simulink model "Citation_2015a"  (R2015a)
settings: Solver=ode5  StartTime=0.0  StopTime=inf  FixedStep=0.01  RelTol=1e-3
InitFcn:
  | initcit
values from neighbouring files (symbols this model uses):
  aeroinit = [dp_ini;inicoef('CX0');inicoef('CXa');inicoef('CXa2');inicoef('CXq')     ;inicoef('CXde');inicoef('CY0');inicoef('CYB');inicoef('CYp');inicoef('CYr')     ;inicoef('CYda');inicoef('CYdr');inicoef('CZ0');inicoef('CZa');inicoef('CZq')     ;inicoef('CZde');inicoef('Cl0');inicoef('ClB');inicoef('Clp');inicoef('Clr')     ;inicoef('Clda');inicoef('Cldr');inicoef('Cm0');inicoef('Cma');inicoef('Cmq')     ; ...(+113 chars)    [initcit.m]
  Clda_thresh = 3.410e-2/2    (= 0.01705)    [initcit.m]
  h_l_old = zeros(6,sample_size)    [initcit.m]
  h_m_old = zeros(4,sample_size)    [initcit.m]
  h_n_old = zeros(6,sample_size)    [initcit.m]
  h_X_old = zeros(5,sample_size)    [initcit.m]
  h_Y_old = zeros(6,sample_size)    [initcit.m]
  h_Z_old = zeros(4,sample_size)    [initcit.m]
  I = [massinit(5),0, -massinit(8);0, massinit(6),0;-massinit(8),0, massinit(7)]    [initcit.m]
  p_l = [inicoef('Cl0');inicoef('ClB');inicoef('Clp');inicoef('Clr')     ;inicoef('Clda');inicoef('Cldr')].*ones(6,sample_size)    [initcit.m]
  p_m = [inicoef('Cm0');inicoef('Cma');inicoef('Cmq')     ;inicoef('Cmde')].*ones(4,sample_size)    [initcit.m]
  p_n = [inicoef('Cn0');inicoef('CnB');inicoef('Cnp');inicoef('Cnr')     ;inicoef('Cnda');inicoef('Cndr')].*ones(6,sample_size)    [initcit.m]
  p_X = [inicoef('CX0');inicoef('CXa');inicoef('CXa2');inicoef('CXq')     ;inicoef('CXde')].*ones(5,sample_size)    [initcit.m]
  p_Y = [inicoef('CY0');inicoef('CYB');inicoef('CYp');inicoef('CYr')     ;inicoef('CYda');inicoef('CYdr')].*ones(6,sample_size)    [initcit.m]
  p_Z = [inicoef('CZ0');inicoef('CZa');inicoef('CZq')     ;inicoef('CZde')].*ones(4,sample_size)    [initcit.m]
  Pcov_l = 10000*eye(6)    [initcit.m]
  Pcov_m = 10000*eye(4)    [initcit.m]
  Pcov_n = 10000*eye(6)    [initcit.m]
  Pcov_X = 10000*eye(5)    [initcit.m]
  Pcov_Y = 10000*eye(6)    [initcit.m]
  Pcov_Z = 10000*eye(4)    [initcit.m]
  replay = 0    [initcit.m]
  T0 = 288.15    [rho_test.m]
  timeend = inputsim.data{1}.Values.Time(end)    [initcit.m]
  Vw915 = 0    [initcit.m]
  winddir = 45*(pi/180)    (= 0.785398163397)    [initcit.m]
  x0 = []    [cessnac550_3d_sfnc.m]    (also in sfunxyauto.m)
  y_l = zeros(1,sample_size)    [initcit.m]
  y_l_est_old = zeros(size(y_l))    [initcit.m]
  y_m = zeros(1,sample_size)    [initcit.m]
  y_m_est_old = zeros(size(y_m))    [initcit.m]
  y_n = zeros(1,sample_size)    [initcit.m]
  y_n_est_old = zeros(size(y_n))    [initcit.m]
  y_X = zeros(1,sample_size)    [initcit.m]
  y_X_est_old = zeros(size(y_X))    [initcit.m]
  y_Y = zeros(1,sample_size)    [initcit.m]
  y_Y_est_old = zeros(size(y_Y))    [initcit.m]
  y_Z = zeros(1,sample_size)    [initcit.m]
  y_Z_est_old = zeros(size(y_Z))    [initcit.m]
undefined symbols (not defined in the file or in its folder): chord, cv1, cv2, cv3, cv4, deltagmax1, deltagmax2, deltagmax3, deltagmax4, Deng, ealphag, ealphas, g0, hDME, hGS, kt1, kt2, kt3, lh, massinit, matbuaf, matdaf, matdam, matdbbf, matdeaf, matdgaf, matdqaf, matduaf, matdwaw, matedhr, mateif, matelhr, matemhr, matemv1, matemv2, matemve, matetam, mateuaf, matfaaf, matfaxl, matff, matibaf, matibmh, matipaf, matipmh, matiraf, matiuaf, matiwaf, matlaf, matlam, matleaf, matleam, matlgaf, matlqaf, matluaf, matmaaf, matmaam, matmaf, matmam, matmbbf ... (+74)
undefined symbols (not defined in the file): matibb
libraries: simulink x13, templibrary x6, vrlib x1
(part 1 of 7)
settings Model: ExtModeTrigMode=oneshot  ExtModeArmWhenConnect=off  Creator=laurensvaneykeren  LastModifiedBy=Jelle
settings DataIOCC: LimitDataPoints=off  SignalLoggingName=sigsOut
settings OptimizationCC: BooleanDataType=off  ExpressionDepthLimit=2147483647
settings DebuggingCC: SaveWithParameterizedLinksMsg=none  UnderspecifiedInitializationDetection=Classic  MergeDetectMultiDrivingBlocksExec=none  SignalResolutionControl=TryResolveAllWithWarning  MultiTaskDSMMsg=warning  MultiTaskCondExecSysMsg=none  FcnCallInpInsideContextMsg=EnableAllAsWarning  StateNameClashWarn=warning
settings HardwareCC: TargetUnknown=on
settings RTWCC: SystemTargetFile=grt_malloc.tlc  GenCodeOnly=on  TemplateMakefile=grt_malloc_default_tmf
settings GRTTargetCC: GeneratePreprocessorConditionals=Use local settings  CombineOutputUpdateFcns=off  GRTInterface=on  UseMalloc=on

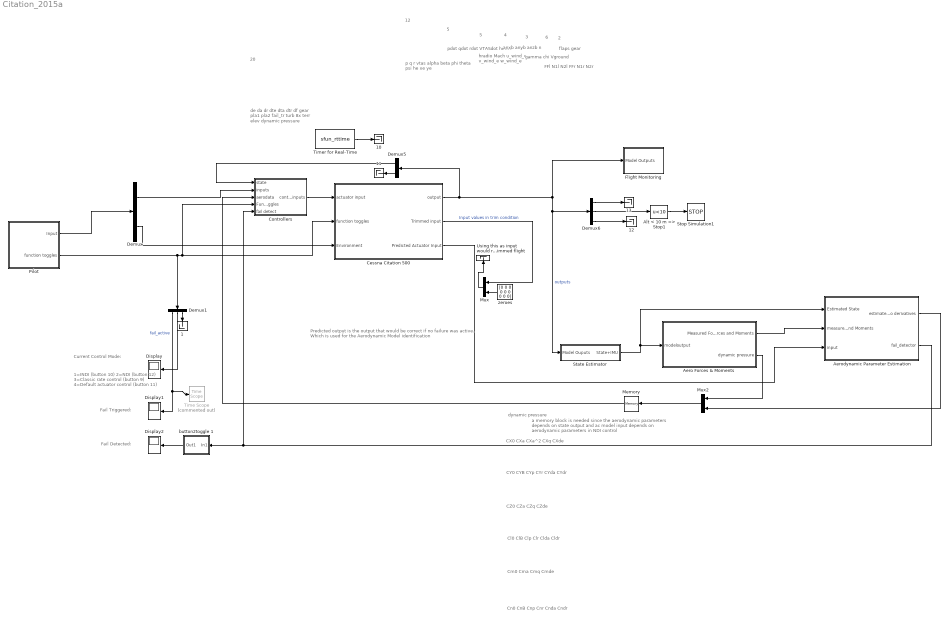
== system Citation_2015a ==
  note: a memory block is needed since the aerodynamic parameters depends on state output and ac model input depends on aerodynamic parameters in NDI control
  note: Predicted output is the output that would be correct if no failure was active.
      | Which is used for the Aerodynamic Model identification
  note: de
      | da
      | dr
      | dte
      | dta
      | dtr
      | df
      | gear
      | pla1
      | pla2
      | fail_tr
      | turb 8x
      | terr elev
      | dynamic pressure
  note: p
      | q
      | r
      | vtas
      | alpha
      | beta
      | phi
      | theta
      | psi
      | he
      | xe
      | ye
  note: pdot
      | qdot
      | rdot
      | VTASdot
      | hedot
  note: hradio
      | Mach
      | u_wind_e
      | v_wind_e
      | w_wind_e
  note: anxb
      | anyb
      | anzb
      | n
  note: gamma
      | chi
      | Vground
  note: flaps
      | gear
  note: FFl
      | N1l
      | N2l
      | FFr
      | N1r
      | N2r
  note: 12
  note: 5
  note: 5
  note: 4
  note: 3
  note: 6
  note: 2
  note: 20
  note: Cn0
      | CnB
      | Cnp
      | Cnr
      | Cnda
      | Cndr
  note: CZ0
      | CZa
      | CZq
      | CZde
  note: Cm0
      | Cma
      | Cmq
      | Cmde
  note: CY0
      | CYB
      | CYp
      | CYr
      | CYda
      | CYdr
  note: Cl0
      | ClB
      | Clp
      | Clr
      | Clda
      | Cldr
  note: CX0
      | CXa
      | CXa^2
      | CXq
      | CXde
  note: dynamic pressure
  note: Current Control Mode:
  note: 1=INDI (button 10)
      | 2=NDI (button 12)
      | 3=Classic rate control (button 9)
      | 4=Default actuator control (button 11)
  note: Fail Triggered:
  note: Fail Detected:
  {1,10..13} (5 alike) : Terminator
  "Aero Forces & Moments " : Subsystem
  Aerodynamic Parameter Estimation : Subsystem
  Alt < 10 m => Stop1 : Fcn  Expr=u<10
  Cessna Citation 500 : Subsystem  mask(Citation Aircraft Model){trimdatafile=example.tri}
      mask prompts: trimdatafile "Trim Condition"
      mask init:
      | initcit;
      mask Display:
      | image(imread('Citation.jpg'))
      | port_label('input', 1, 'Inputs')
      | port_label('input', 2, 'Function Toggles')
      | port_label('input', 3, 'Environment')
      | port_label('output', 1, 'Outputs')
      | port_label('output', 2, 'Trim inputs')
      | port_label('output', 3, 'Predicted control input')
  Controllers : Subsystem
  Demux : Demux  Outputs=[10 9]
  Demux1 : Demux  Outputs=[1 1 2]
  Demux5 : Demux  Outputs=[17 20]
  Demux6 : Demux  Outputs=[9 1 27]
  Display : Display
  Display1 : Display
  Display2 : Display
  Flight Monitoring : Subsystem
  Memory : Memory  X0=aeroinit
  Mux : Mux  Inputs=2
  Mux2 : Mux  Inputs=2
  Pilot : Subsystem
  "State Estimator " : Subsystem
  Stop Simulation1 : Stop
  Time Scope : TimeScope  Commented=on  DefaultConfigurationName=spbscopes.TimeScopeBlockCfg
  Timer for Real-Time : S-Function  FunctionName=sfun_rttime  Parameters=1  SFunctionDeploymentMode=off  EnableBusSupport=off
  Using this as input would result in trimmed flight : Terminator
  button2toggle 1 : Subsystem
  zeroes : Constant  Value=[0 0 0 0 0 0 0 0 0]
  wires:
  Demux/1 -> Controllers/2(inputs)
  Pilot/1(Input) -> Demux/1
  Cessna Citation 500/1(output) -> Demux6/1, "State Estimator "/1(Model Ouputs), Flight Monitoring/1(Model Outputs), Demux5/1  "outputs"
  Demux/2 -> Cessna Citation 500/3(Environment)
  Cessna Citation 500/2(Trimmed input) -> Mux/1  "Input values in trim condition"
  zeroes/1 -> Mux/2
  Mux/1 -> Using this as input would result in trimmed flight/1
  "State Estimator "/1(State+IMU) -> Aerodynamic Parameter Estimation/1("Estimated State "), "Aero Forces & Moments "/1(modeloutput)
  Cessna Citation 500/3(Predicted Actuator Input) -> Aerodynamic Parameter Estimation/3("input ")
  "Aero Forces & Moments "/1(Measured Forces and Moments) -> Aerodynamic Parameter Estimation/2("measured forces and Moments ")
  Aerodynamic Parameter Estimation/1(estimated aero derivatives) -> Mux2/2
  "Aero Forces & Moments "/2("dynamic pressure ") -> Mux2/1
  Mux2/1 -> Memory/1
  Memory/1 -> Controllers/3(aerodata)
  Timer for Real-Time/1 -> 10/1
  Aerodynamic Parameter Estimation/2(fail_detector) -> Controllers/5(fail detect), button2toggle 1/1(In1)
  Demux5/2 -> 11/1
  Demux5/1 -> Controllers/1(state)
  Controllers/1(control inputs) -> Cessna Citation 500/1(actuator input)
  Demux6/3 -> 12/1
  Demux6/1 -> 13/1
  Demux6/2 -> Alt < 10 m => Stop1/1
  Alt < 10 m => Stop1/1 -> Stop Simulation1/1
  Pilot/2(function toggles) -> Controllers/4("Function Toggles "), Cessna Citation 500/2("function toggles "), Demux1/1
  Demux1/1 -> Time Scope/1, Display1/1  "fail_active"
  Demux1/2 -> Display/1
  button2toggle 1/1(Out1) -> Display2/1
  Demux1/3 -> 1/1

== system Citation_2015a/Aero Forces & Moments  ==
  note: Kinematic Force Coeffient determination
  note: anxb
      | anyb
      | anzb
      | n
  note: hradio
      | Mach
      | u_wind_e
      | v_wind_e
      | w_wind_e
  note: p
      | q
      | r
      | vtas
      | alpha
      | beta
      | phi
      | theta
      | psi
      | he
      | xe
      | ye
  note: gamma
      | chi
      | Vground
  note: pdot
      | qdot
      | rdot
      | VTASdot
      | hedot
  note: FFl
      | N1l
      | N2l
      | FFr
      | N1r
      | N2r
  note: flaps
      | gear
  note: 6
  note: 5
  note: 12
  note: 3
  note: 5
  note: 4
  note: 2
  note: CX
      | CY
      | CZ
      | Cl
      | Cm
      | Cn
  modeloutput : Inport
  Aerodynamic Force Components : Subsystem
  Aerodynamic Moment Components : Subsystem
  Calculate Dynamic Pressure : Subsystem
  Mux : Mux  Inputs=2
  Measured Forces and Moments : Outport
  "dynamic pressure " : Outport  Port=2
  wires:
  Aerodynamic Force Components/1(Out1) -> Mux/1
  modeloutput/1 -> Calculate Dynamic Pressure/1(In1), Aerodynamic Moment Components/1("State "), Aerodynamic Force Components/1("model output ")
  Calculate Dynamic Pressure/1(Out1) -> "dynamic pressure "/1, Aerodynamic Moment Components/2("Dynamic Pressure "), Aerodynamic Force Components/2(dynamic pressure)
  Aerodynamic Moment Components/1(Out1) -> Mux/2
  Mux/1 -> Measured Forces and Moments/1

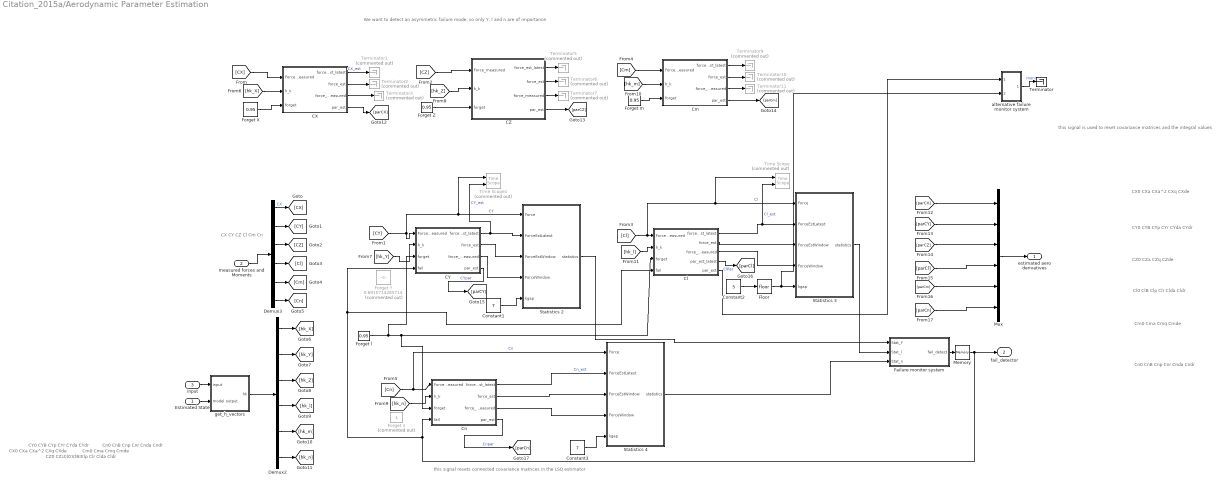
== system Citation_2015a/Aerodynamic Parameter Estimation ==
  note: this signal is used to reset covariance matrices and the integral values
  note: this signal resets connected covariance matrices in the LSQ estimator
  note: We want to detect an asymmetric failure mode, so only Y, l and n are of importance
  note: CX
      | CY
      | CZ
      | Cl
      | Cm
      | Cn
  note: Cm0
      | Cma
      | Cmq
      | Cmde
  note: Cn0
      | CnB
      | Cnp
      | Cnr
      | Cnda
      | Cndr
  note: CY0
      | CYB
      | CYp
      | CYr
      | CYda
      | CYdr
  note: CZ0
      | CZa
      | CZq
      | CZde
  note: CX0
      | CXa
      | CXa^2
      | CXq
      | CXde
  note: Cl0
      | ClB
      | Clp
      | Clr
      | Clda
      | Cldr
  note: Cl0
      | ClB
      | Clp
      | Clr
      | Clda
      | Cldr
  note: CY0
      | CYB
      | CYp
      | CYr
      | CYda
      | CYdr
  note: Cm0
      | Cma
      | Cmq
      | Cmde
  note: CX0
      | CXa
      | CXa^2
      | CXq
      | CXde
  note: CZ0
      | CZa
      | CZq
      | CZde
  note: Cn0
      | CnB
      | Cnp
      | Cnr
      | Cnda
      | Cndr
  "Estimated State " : Inport
  "measured forces and Moments " : Inport  Port=2
  "input " : Inport  Port=3
  CX : Subsystem
  CY : Subsystem
  CZ : Subsystem
  Cl : Subsystem
  Cm : Subsystem
  Cn : Subsystem
  Constant1 : Constant  Value=7
  Constant2 : Constant  Value=5
  Constant3 : Constant  Value=7
  Demux2 : Demux  Outputs=[5 6 4 6 4 6]
  Demux3 : Demux  Outputs=[1 1 1 1 1 1]
  "Failure monitor system " : Subsystem
  Floor : Rounding
  Forget X : Constant  Value=0.95
  Forget Y : Constant  Commented=on  Value=0.6910714285714
  Forget Z : Constant  Value=0.95
  Forget l : Constant  Value=0.95
  Forget m : Constant  Value=0.95
  Forget n : Constant  Commented=on
  Memory : Memory
  Mux : Mux  Inputs=6
  Statistics 2 : Subsystem
  Statistics 3 : Subsystem
  Statistics 4 : Subsystem
  Terminator : Terminator
  Terminator{1..3,5..7,9..11} (9 alike) : Terminator  Commented=on
  Time Scope : TimeScope  Commented=on  DefaultConfigurationName=spbscopes.TimeScopeBlockCfg  NumInputPorts=2
  Time Scope1 : TimeScope  Commented=on  DefaultConfigurationName=spbscopes.TimeScopeBlockCfg  NumInputPorts=2
  alternative failure monitor system : Subsystem
  get_h_vectors : Subsystem
  estimated aero derivatives : Outport
  fail_detector : Outport  Port=2
  wires:
  "input "/1 -> get_h_vectors/1(input)
  "Estimated State "/1 -> get_h_vectors/2(model output)
  get_h_vectors/1(hk) -> Demux2/1
  "measured forces and Moments "/1 -> Demux3/1
  Demux3/2 -> [CY]
  CX/4(par_est) -> [parCX]
  Forget X/1 -> CX/3(forget)
  Forget Z/1 -> CZ/3(forget)
  Forget l/1 -> CY/3(forget), Cn/3(forget), Cl/3(forget)
  Forget m/1 -> Cm/3(forget)
  CY/1(force_est_latest) -> Time Scope1/2, Statistics 2/2(ForceEstLatest)  "CY_est"
  CY/2(force_est) -> Statistics 2/3(ForceEstWindow)
  CY/3(force_measured) -> Statistics 2/4(ForceWindow)
  Constant1/1 -> Statistics 2/5("kgap ")
  Cl/1(force_est_latest) -> Time Scope/2, Statistics 3/2(ForceEstLatest)  "Cl_est"
  Cl/2(force_est) -> Statistics 3/3(ForceEstWindow)
  Cl/3(force_measured) -> Statistics 3/4(ForceWindow)
  Constant2/1 -> Floor/1
  Cn/1(force_est_latest) -> Statistics 4/2(ForceEstLatest)  "Cn_est"
  Cn/2(force_est) -> Statistics 4/3(ForceEstWindow)
  Constant3/1 -> Statistics 4/5("kgap ")
  Demux3/1 -> [CX]  "CX"
  [CX] -> CX/1(Force_measured)
  [CY] -> CY/1(Force_measured), Time Scope1/1, Statistics 2/1(Force)  "CY"
  Demux3/3 -> [CZ]
  [CZ] -> CZ/1(Force_measured)
  Demux3/4 -> [Cl]
  [Cl] -> Time Scope/1, Statistics 3/1(Force), Cl/1(Force_measured)  "Cl"
  Demux3/5 -> [Cm]
  [Cm] -> Cm/1(Force_measured)
  Demux3/6 -> [Cn]
  [Cn] -> Statistics 4/1(Force), Cn/1(Force_measured)  "Cn"
  Demux2/1 -> [hk_X]
  Demux2/2 -> [hk_Y]
  Demux2/3 -> [hk_Z]
  Demux2/4 -> [hk_l]
  Demux2/5 -> [hk_m]
  Demux2/6 -> [hk_n]
  [hk_X] -> CX/2(h_k)
  [hk_Y] -> CY/2(h_k)
  [hk_Z] -> CZ/2(h_k)
  [hk_l] -> Cl/2(h_k)
  [hk_m] -> Cm/2(h_k)
  [hk_n] -> Cn/2(h_k)
  Cn/3(force_measured) -> Statistics 4/4(ForceWindow)
  CX/1(force_est_latest) -> Terminator1/1  "CX_est"
  CX/2(force_est) -> Terminator2/1
  CX/3(force_measured) -> Terminator3/1
  CY/4(par_est) -> [parCY]  "CYpar"
  CZ/2(force_est) -> Terminator6/1
  CZ/3(force_measured) -> Terminator7/1
  CZ/1(force_est_latest) -> Terminator5/1
  Cm/1(force_est_latest) -> Terminator9/1
  Cm/2(force_est) -> Terminator10/1
  Cm/3(force_measured) -> Terminator11/1
  Cm/4(par_est) -> [parCm]
  Statistics 4/1(statistics) -> "Failure monitor system "/3(Stat_n)
  Statistics 3/1(statistics) -> "Failure monitor system "/2(Stat_l)
  Statistics 2/1(statistics) -> "Failure monitor system "/1(Stat_Y)
  CZ/4(par_est) -> [parCZ]
  Cl/4(par_est_latest) -> [parCl]  "ClPar"
  Cn/4(par_est) -> [parCn]  "Cnpar"
  [parCX] -> Mux/1
  [parCY] -> Mux/2
  [parCZ] -> Mux/3
  [parCl] -> Mux/4
  [parCm] -> Mux/5
  [parCn] -> Mux/6
  Mux/1 -> estimated aero derivatives/1
  Floor/1 -> alternative failure monitor system/2(In3), Statistics 3/5("kgap ")
  Cl/5(par_est) -> alternative failure monitor system/1(In2)
  "Failure monitor system "/1(fail_detect) -> Memory/1
  Memory/1 -> fail_detector/1, Cl/4("fail "), CY/4(fail), Cn/4("fail ")
  alternative failure monitor system/1(Out1) -> Terminator/1  "moni"

== system Citation_2015a/Cessna Citation 500 ==
  note: this is the actuator input that is always without failure
  note: p
      | q
      | r
      | vtas
      | alpha
      | beta
      | phi
      | theta
      | psi
      | he
      | xe
      | ye
  note: de
      | da
      | dr
      | dte
      | dta
      | dtr
      | df
      | gear
      | pla1
      | pla2
  note: pdot
      | qdot
      | rdot
      | VTASdot
      | hedot
  note: hradio
      | Mach
      | u_wind_e
      | v_wind_e
      | w_wind_e
  note: anxb
      | anyb
      | anzb
      | n
  note: gamma
      | chi
      | Vground
  note: turb 8x
      | terr_elev
  note: flaps
      | gear
  note: de
      | da
      | dr
      | dte
      | dta
      | dtr
      | df
      | gear
      | pla1
      | pla2
  note: FFl
      | N1l
      | N2l
      | FFr
      | N1r
      | N2r
  note: fail_aileron
  actuator input : Inport
  "function toggles " : Inport  Port=2
  Environment : Inport  Port=3
  Actuators : Subsystem
  Citation model DASMAT : Subsystem
  Control Inputs : TimeScope  Commented=on  DefaultConfigurationName=spbscopes.TimeScopeBlockCfg  NumInputPorts=3
  Demux : Demux  Outputs=[1 3]
  Demux1 : Demux  Outputs=[1 1 1 7]
  Demux4 : Demux  Outputs=[8 2]
  Gain : Gain  Commented=on  Gain=180/pi
  Gain1 : Gain  Commented=on  Gain=180/pi
  Gain2 : Gain  Commented=on  Gain=180/pi
  Mux1 : Mux  Inputs=7
  Mux2 : Mux  Inputs=2
  Terminator : Terminator
  Terminator1 : Terminator
  trim conditions : Subsystem
  ua sel : Selector  IndexOptions=Index vector (dialog)  Indices=[5 6]  OutputSizes=1
  xdot sel : Selector  IndexOptions=Index vector (dialog)  Indices=[1 2 3 4 10]  OutputSizes=1
  yacc sel : Selector  IndexOptions=Index vector (dialog)  Indices=[4 5 6 15]  OutputSizes=1
  yair sel : Selector  IndexOptions=Index vector (dialog)  Indices=[6 9 22 23 24]  OutputSizes=1
  yfp sel : Selector  IndexOptions=Index vector (dialog)  Indices=[1 2 15]  OutputSizes=1
  ypp sel : Selector  IndexOptions=Index vector (dialog)  Indices=[2 3 4 13 14 15]  OutputSizes=1
  output : Outport
  Trimmed input : Outport  Port=2
  Predicted Actuator Input : Outport  Port=3
  wires:
  Mux1/1 -> output/1
  Citation model DASMAT/1(x) -> Mux1/1
  Demux4/1 -> Citation model DASMAT/1(ua), ua sel/1
  Demux4/2 -> Citation model DASMAT/2(ut)
  Citation model DASMAT/3(yair) -> yair sel/1
  yair sel/1 -> Mux1/3
  Citation model DASMAT/2(xdot) -> xdot sel/1
  xdot sel/1 -> Mux1/2
  yacc sel/1 -> Mux1/4
  Citation model DASMAT/4(yacc) -> yacc sel/1
  yfp sel/1 -> Mux1/5
  Citation model DASMAT/5(yfp) -> yfp sel/1
  trim conditions/1(ua) -> Mux2/1
  trim conditions/2(ut) -> Mux2/2
  Mux2/1 -> Trimmed input/1
  ua sel/1 -> Mux1/7
  Citation model DASMAT/6(ypp) -> ypp sel/1
  ypp sel/1 -> Mux1/6
  Actuators/2(Actuator_pred) -> Predicted Actuator Input/1
  Environment/1 -> Citation model DASMAT/3(Environment)
  Demux1/1 -> Gain/1  "de true"
  Demux1/2 -> Gain1/1  "da true"
  Demux1/3 -> Gain2/1  "dr true"
  Demux1/4 -> Terminator/1
  actuator input/1 -> Actuators/1(In)  "actuator_input"
  Demux/1 -> Actuators/2("failure toggle ")
  "function toggles "/1 -> Demux/1
  Demux/2 -> Terminator1/1
  Actuators/1(Actuator_True) -> Demux1/1, Demux4/1
  Gain/1 -> Control Inputs/1
  Gain1/1 -> Control Inputs/2
  Gain2/1 -> Control Inputs/3

== system Citation_2015a/Controllers ==
  note: map joystick inputs to reference rotational rates
  note: This signal resets the integral values of all connected PIDs
      | Resets when manually changing the control mode and when failure state changes.
  note: 1=INDI (button 10)
      | 2=NDI (button 12)
      | 3=Classic rate control (button 9)
      | 4=Default actuator control (button 11)
  note: Aerodata Description
  note: [1]
  note: p
      | q
      | r
      | vtas
      | alpha
      | beta
      | phi
      | theta
      | psi
      | he
      | xe
      | ye
  note: de
      | da
      | dr
      | dte
      | dta
      | dtr
      | df
      | gear
      | pla1
      | pla2
  note: CX0
      | CXa
      | CXa^2
      | CXq
      | CXde
  note: Cm0
      | Cma
      | Cmq
      | Cmde
  note: CY0
      | CYB
      | CYp
      | CYr
      | CYda
      | CYdr
  note: CZ0
      | CZa
      | CZq
      | CZde
  note: Cn0
      | CnB
      | Cnp
      | Cnr
      | Cnda
      | Cndr
  note: dynamic pressure
  note: Cl0
      | ClB
      | Clp
      | Clr
      | Clda
      | Cldr
  note: [2:6]
  note: [7:12]
  note: [13:16]
  note: [17:22]
  note: [23:26]
  note: [27:32]
  state : Inport
  inputs : Inport  Port=2
  aerodata : Inport  Port=3
  "Function Toggles " : Inport  Port=4
  fail detect : Inport  Port=5
  "A/T " : Gain  Gain=[1 1 1 1 1 1 1 1 1 1]  SaturateOnIntegerOverflow=on  OutDataTypeStr=Inherit: Same as input  ParamDataTypeStr=Inherit: Same as input
  ANDI rotational rate controller : Subsystem
  Classical rotational rate control : Subsystem
  Constant : Constant
  Constant1 : Constant  Value=0
  Constant3 : Constant  Commented=on  Value=aeroinit
  Default Actuator Control : Subsystem
  Demux1 : Demux  Outputs=[12 5]
  Demux2 : Demux
  Display1 : Display
  Gain : Gain
  Generate Integral reset pulse : Subsystem
  INDI rotational rate controller : Subsystem
  Input to omega_ref (Beta feedback included) : Subsystem
  Memory : Memory  X0=zeros(5,1)
  Multiply : Product
  Multiport Switch : MultiPortSwitch  Inputs=4
  Switch : Switch  Criteria=u2 > Threshold
  Terminator1 : Terminator
  add controller outputs to pilot inputs : Sum  Inputs=|+|+|  SaturateOnIntegerOverflow=on
  auto throttle : Subsystem
  control inputs : Outport
  wires:
  inputs/1 -> Default Actuator Control/2(inputs), Input to omega_ref (Beta feedback included)/1(Input)
  add controller outputs to pilot inputs/1 -> control inputs/1
  auto throttle/1(controller output) -> Multiply/2
  Multiply/1 -> add controller outputs to pilot inputs/1
  Multiport Switch/1 -> auto throttle/2(inputs), "A/T "/1
  "A/T "/1 -> add controller outputs to pilot inputs/2
  ANDI rotational rate controller/1(control input) -> Multiport Switch/3
  Default Actuator Control/1(control inputs) -> Multiport Switch/5
  aerodata/1 -> ANDI rotational rate controller/3(aero data), INDI rotational rate controller/5(airdata)
  Input to omega_ref (Beta feedback included)/1(omega_ref) -> Classical rotational rate control/1(inputs), INDI rotational rate controller/1(Inputs), ANDI rotational rate controller/1(inputs)
  Classical rotational rate control/1(control inputs) -> Multiport Switch/4
  Gain/1 -> ANDI rotational rate controller/2(A/C state), Default Actuator Control/1(state), INDI rotational rate controller/2(state), Classical rotational rate control/2(state), auto throttle/1(state), Input to omega_ref (Beta feedback included)/2(state)
  state/1 -> Demux1/1
  Demux1/1 -> Gain/1  "x"
  Demux1/2 -> Memory/1  "xdot"
  INDI rotational rate controller/1(Out1) -> Multiport Switch/2
  Memory/1 -> INDI rotational rate controller/4(xdot)
  Generate Integral reset pulse/1(reset_pulse) -> ANDI rotational rate controller/4(int reset), Classical rotational rate control/3(int reset), INDI rotational rate controller/3(int reset)
  fail detect/1 -> Generate Integral reset pulse/2(fail detect)
  Demux2/2 -> Generate Integral reset pulse/1(mode toggle), Multiport Switch/1, Display1/1
  "Function Toggles "/1 -> Demux2/1
  Demux2/1 -> Terminator1/1
  Demux2/3 -> Generate Integral reset pulse/3(manual_reset)
  Demux2/4 -> Switch/2  "autothrottle toggle"
  Switch/1 -> Multiply/1
  Constant/1 -> Switch/1
  Constant1/1 -> Switch/3

== system Citation_2015a/Flight Monitoring ==
  note: pdot
      | qdot
      | rdot
      | VTASdot
      | hedot
  note: hradio
      | Mach
      | u_wind_e
      | v_wind_e
      | w_wind_e
  note: gamma
      | chi
      | Vground
  note: 5
  note: anxb
      | anyb
      | anzb
      | n
  note: 2
  note: 4
  note: 3
  note: flaps
      | gear
  note: 6
  note: p
      | q
      | r
      | vtas
      | alpha
      | beta
      | phi
      | theta
      | psi
      | he
      | xe
      | ye
  note: FFl
      | N1l
      | N2l
      | FFr
      | N1r
      | N2r
  Model Outputs : Inport
  {1..10} (10 alike) : Terminator
  3D Display : Subsystem
  3D Graph : S-Function  Commented=on  LoadFcn=if exist('sfun3d','file'), sfun3d([],[],[],'LoadBlock'); end  FunctionName=sfun3d  Parameters=ax,T,np,cp,gd,ls,mk,mx,hd,tb  SFunctionDeploymentMode=off  EnableBusSupport=off  mask(3D Graph){np=1, ax=[-2000 7000 -100 15000 1500 2500], mx=1e8, T=0.01, cp=[1 1 0.5], gd=on, hd=on, tb=on, ls=-, mk=none}
      mask prompts: np "Number of moving points (lines)"; ax "Range: [xmin xmax  ymin ymax zmin zmax]"; mx "Max number of points in each line"; T "Sampling Time"; cp "Camera position (use [0 0 1] for 2D XY view)"; gd "Grid (on|off)"; hd "HeadMarkers (on|off)"; tb "Toolbar (on|off)"; ls "LineStyle"; mk "LineMarker"
      mask help:
      | This block plots the position of several points in the XYZ space. The input contains the coordinates of all the points (x1,y1,z1,x2,y2,z2,...).
      | The number of moving points (lines), the XYZ ranges, sampling time, camera position, and grid (among other things) can be set as mask parameters.
      settings: CopyFcn=if exist('sfun3d','file'), sfun3d([],[],[],'CopyBlock'); end  DeleteFcn=if exist('sfun3d','file'), sfun3d([],[],[],'DeleteBlock'); end  NameChangeFcn=if exist('sfun3d','file'), sfun3d([],[],[],'NameChange'); end
      mask Help:
      | This block plots the position of several points in the XYZ space. The input contains the coordinates of all the points (x1,y1,z1,x2,y2,z2,...).
      | The number of moving points (lines), the XYZ ranges, sampling time, camera position, and grid (among other things) can be set as mask parameters.
      mask TypeOptions ls: - | -- | : | -. | none
      mask TypeOptions mk: none | . | + | o | * | x | square | diamond | v | ^ | > | < | pentagram | hexagram
      mask Display: plot([.05 .95 .95 .05 .05],[.45 .45 .95 .95 .45], 0.5+cos(0:0.1:2*pi)*0.3,0.7+sin(0:0.1:2*pi)*0.2)
  Clock : Clock
  Demux : Demux  Outputs=3
  Demux1 : Demux  Outputs=[6 1 1 1 17 1 1 9]
  Demux2 : Demux  Outputs=[3 1 1 2 1 1 1 8 1 1 1 16]
  Demux3 : Demux  Outputs=[9 1 1 1 25]
  Demux4 : Demux  Outputs=2
  Gain{,1..4} (5 alike) : Gain  Gain=180/pi
  Mux1 : Mux  Inputs=3
  Position : Display
  Sum : Sum  Inputs=|-+
  Time Scope{,2..3,5} (4 alike) : TimeScope  Commented=on  DefaultConfigurationName=spbscopes.TimeScopeBlockCfg  NumInputPorts=3
  Time Scope1 : TimeScope  Commented=on  DefaultConfigurationName=spbscopes.TimeScopeBlockCfg
  Time Scope4 : TimeScope  Commented=on  DefaultConfigurationName=spbscopes.TimeScopeBlockCfg
  Vtas : templibrary/XY Graph  Autoscale  Commented=on  xmin=-1  xmax=1  ymin=-1  ymax=1  st=0
  X : templibrary/XY Graph  Autoscale  xmin=-1  xmax=1  ymin=-1  ymax=1  st=0
  Y : templibrary/XY Graph  Autoscale  Commented=on  xmin=-1  xmax=1  ymin=-1  ymax=1  st=0
  Z : templibrary/XY Graph  Autoscale  Commented=on  xmin=-1  xmax=1  ymin=-1  ymax=1  st=0
  altitude : templibrary/XY Graph  Autoscale  Commented=on  xmin=-1  xmax=1  ymin=-1  ymax=1  st=0.01
      link override S-Function: Parameters="[xmin xmax ymin ymax],  st"
  flight path : Display
  gamma : templibrary/XY Graph  Autoscale  Commented=on  xmin=-1  xmax=1  ymin=-1  ymax=1  st=0
  heading : Display
  "phi " : Display
  wires:
  Demux2/5 -> Sum/2  "theta"
  Demux2/10 -> Time Scope/2
  Demux1/2 -> Gain4/1, 3D Display/1(roll)  "Phi"
  Demux1/3 -> 3D Display/2(pitch)  "theta"
  Clock/1 -> Z/1, Y/1, X/1, gamma/1, altitude/1, Vtas/1
  Demux2/8 -> 6/1
  Demux2/2 -> Vtas/2, Time Scope1/1  "vtas"
  Demux2/1 -> Demux/1
  Demux2/6 -> 9/1
  Demux3/1 -> 7/1
  Demux2/12 -> 5/1
  Demux2/7 -> altitude/2  "h"
  Demux2/3 -> Sum/1  "alpha"
  Demux3/4 -> Time Scope3/2, Y/2, Mux1/2  "Y"
  Demux1/1 -> 1/1
  Demux1/4 -> 3D Display/3(yaw)  "Psi"
  Demux1/5 -> 2/1
  Demux3/3 -> Time Scope3/1, X/2, Mux1/1  "X"
  Sum/1 -> Gain/1  "gamma"
  Mux1/1 -> Position/1, 3D Graph/1
  Demux3/2 -> Time Scope3/3, Z/2, Mux1/3  "Z"
  Demux2/9 -> Time Scope/1
  Demux2/11 -> Time Scope/3
  Demux3/5 -> 8/1
  Gain/1 -> gamma/2  "gamma[deg]"
  Demux2/4 -> Demux4/1, 4/1
  Model Outputs/1 -> Demux1/1, Demux3/1, Demux2/1
  Demux/2 -> Time Scope2/2  "q"
  Demux1/6 -> Gain2/1
  Demux1/7 -> Gain1/1
  Gain1/1 -> heading/1, Time Scope4/1, Time Scope5/2  "heading"
  Gain2/1 -> flight path/1, Time Scope5/1  "gamma"
  Demux4/2 -> Gain3/1
  Gain3/1 -> Time Scope5/3  "phi"
  Demux/1 -> Time Scope2/1
  Demux/3 -> Time Scope2/3
  Gain4/1 -> "phi "/1
  Demux1/8 -> 3/1
  Demux4/1 -> 10/1

== system Citation_2015a/Pilot ==
  note: button2toggle toggles between a constant 1 or 0 when an input pulse is given
  note: de
      | da
      | dr
      | dte
      | dta
      | dtr
      | df
      | gear
      | pla1
      | pla2
      | turb 8x
      | terr elev
  note: 1=INDI
      | 2=NDI
      | 3=Classic rate control
      | 4=Default actuator control
  Joystick : Subsystem
  Mux : Mux  Inputs=12
  Mux1 : Mux
  Select new mode : Subsystem
  button2toggle 1 : Subsystem
  button2toggle 2 : Subsystem
  button2toggle 3 : Subsystem
  button2toggle 4 : Subsystem
  button2toggle 5 : Subsystem
  button2toggle 6 : Subsystem
  button2toggle 7 : Subsystem
  da trim : Constant  Value=0
  de trim : Constant  Value=0
  delta flaps : Constant  Value=0
  dr trim : Constant  Value=0
  gear (ON=1/OFF=0) : Constant  Value=0
  terr elev : Constant  Value=0
  turb 8x : Constant  Value=zeros(1,8)
  Input : Outport
  function toggles : Outport  Port=2
  wires:
  Mux/1 -> Input/1
  Joystick/1(delta elevator) -> Mux/1
  Joystick/3(delta rudder) -> Mux/3
  da trim/1 -> Mux/5
  de trim/1 -> Mux/4
  Joystick/2(delta aileron) -> Mux/2
  turb 8x/1 -> Mux/11
  terr elev/1 -> Mux/12
  Joystick/4(Throttle setting) -> Mux/10, Mux/9
  gear (ON=1/OFF=0)/1 -> Mux/8
  dr trim/1 -> Mux/6
  delta flaps/1 -> Mux/7
  Joystick/5("Failure Button ") -> button2toggle 5/Trigger, button2toggle 5/1(In1)
  button2toggle 5/1(Out1) -> Mux1/1
  Joystick/6(NDI Button) -> button2toggle 1/Trigger, button2toggle 1/1(In1)
  Joystick/7(Default Mode button) -> button2toggle 2/Trigger, button2toggle 2/1(In1)
  Joystick/8(Classical rate Mode button) -> button2toggle 3/1(In1), button2toggle 3/Trigger
  Joystick/9(INDI mode button) -> button2toggle 4/Trigger, button2toggle 4/1(In1)
  button2toggle 1/1(Out1) -> Select new mode/1(In1)
  button2toggle 2/1(Out1) -> Select new mode/2(In2)
  button2toggle 3/1(Out1) -> Select new mode/3(In3)
  button2toggle 4/1(Out1) -> Select new mode/4(In4)
  Select new mode/1(Out1) -> Mux1/2
  Mux1/1 -> function toggles/1
  button2toggle 6/1(Out1) -> Mux1/3
  Joystick/10(man_int_reset) -> button2toggle 6/Trigger, button2toggle 6/1(In1)
  Joystick/11("Autothrottle ") -> button2toggle 7/Trigger, button2toggle 7/1(In1)
  button2toggle 7/1(Out1) -> Mux1/4

== system Citation_2015a/State Estimator  ==
  note: It is assumed that the model ouputs are perfect measurements
  Model Ouputs : Inport
  State+IMU : Outport
  wires:
  Model Ouputs/1 -> State+IMU/1

== system Citation_2015a/button2toggle 1 ==
  In1 : Inport
  Constant1 : Constant
  Constant2 : Constant  Value=0
  Memory : Memory  InheritSampleTime=on
  Multiply : Product
  Switch : Switch  Criteria=u2 > Threshold
  Triggered Subsystem : Subsystem  TreatAsAtomicUnit=on
  Out1 : Outport
  wires:
  Constant2/1 -> Switch/1
  Memory/1 -> Switch/2
  Constant1/1 -> Multiply/1
  Multiply/1 -> Switch/3
  In1/1 -> Triggered Subsystem/Trigger, Multiply/2
  Switch/1 -> Triggered Subsystem/1(In1)
  Triggered Subsystem/1(Out1) -> Memory/1, Out1/1

== system Citation_2015a/Aero Forces & Moments /Aerodynamic Force Components ==
  note: Massinit
      | [mass cg? ? ? Ixx Iyy Izz Ixz]
  note: State
  note: accelerations are given in [g]
  note: p
      | q
      | r
      | vtas
      | alpha
      | beta
      | phi
      | theta
      | psi
      | he
      | xe
      | ye
  note: gamma
      | chi
      | Vground
  note: hradio
      | Mach
      | u_wind_e
      | v_wind_e
      | w_wind_e
  note: anxb
      | anyb
      | anzb
      | n
  note: 5
  note: 12
  note: 4
  note: flaps
      | gear
  note: 3
  note: 6
  note: FFl
      | N1l
      | N2l
      | FFr
      | N1r
      | N2r
  note: 5
  note: pdot
      | qdot
      | rdot
      | VTASdot
      | hedot
  note: 2
  "model output " : Inport
  dynamic pressure : Inport  Port=2
  Constant : Constant  Value=massinit
  Demux : Demux  Outputs=[22 3 12]
  Demux2 : Demux  Outputs=[1 7]
  Divide : Product  Inputs=*/
  Gain : Gain  Gain=g0
  Product2 : Product
  Terminator1 : Terminator
  Terminator2 : Terminator
  Terminator4 : Terminator
  Out1 : Outport
  wires:
  Demux/2 -> Gain/1
  Gain/1 -> Product2/1
  dynamic pressure/1 -> Divide/2
  Product2/1 -> Divide/1
  Divide/1 -> Out1/1
  Demux/1 -> Terminator1/1
  Demux/3 -> Terminator2/1
  "model output "/1 -> Demux/1
  Demux2/1 -> Product2/2  "mass"
  Constant/1 -> Demux2/1
  Demux2/2 -> Terminator4/1

== system Citation_2015a/Aero Forces & Moments /Aerodynamic Moment Components ==
  note: p
      | q
      | r
      | vtas
      | alpha
      | beta
      | phi
      | theta
      | psi
      | he
      | xe
      | ye
  note: gamma
      | chi
      | Vground
  note: hradio
      | Mach
      | u_wind_e
      | v_wind_e
      | w_wind_e
  note: anxb
      | anyb
      | anzb
      | n
  note: 5
  note: 12
  note: 4
  note: flaps
      | gear
  note: 3
  note: 6
  note: FFl
      | N1l
      | N2l
      | FFr
      | N1r
      | N2r
  note: 5
  note: pdot
      | qdot
      | rdot
      | VTASdot
      | hedot
  note: 2
  note: Massinit
      | [mass cg? ? ? Ixx Iyy Izz Ixz]
  "State " : Inport
  "Dynamic Pressure " : Inport  Port=2
  Cl : Subsystem
  Cm : Subsystem
  Cn : Subsystem
  Mux : Mux  Inputs=3
  Out1 : Outport
  wires:
  "State "/1 -> Cl/1(model output), Cm/1("model output "), Cn/1(model output)
  "Dynamic Pressure "/1 -> Cn/2(Dynamic Pressure), Cm/2(Dynamic Pressure), Cl/2(Dynamic Pressure)
  Cl/1(Cl) -> Mux/1
  Cn/1(Cn) -> Mux/3
  Cm/1(Cm) -> Mux/2
  Mux/1 -> Out1/1

== system Citation_2015a/Aero Forces & Moments /Calculate Dynamic Pressure ==
  note: Dynamic Pressure
  In1 : Inport
  Calculate Air Density : MATLAB Function  TreatAsAtomicUnit=on
      settings: PermitHierarchicalResolution=ParametersOnly
  Demux : Demux  Outputs=[3 1 33]
  Gain : Gain  Gain=0.5
  Gain1 : Gain  Gain=S
  Product : Product
  Product1 : Product
  Terminator1 : Terminator
  Terminator2 : Terminator
  Out1 : Outport
  wires:
  Product/1 -> Product1/1  "V^2"
  Demux/3 -> Terminator2/1
  Demux/2 -> Product/2, Product/1  "Vtas"
  In1/1 -> Demux/1, Calculate Air Density/1(state)
  Product1/1 -> Gain/1
  Calculate Air Density/1(rho) -> Product1/2  "Rho"
  Demux/1 -> Terminator1/1
  Gain/1 -> Gain1/1
  Gain1/1 -> Out1/1  "0.5*RHO*v^2*S"

== system Citation_2015a/Aerodynamic Parameter Estimation/CX ==
  note: counter is still obsolete
  note: if lambda=1 => no forgetting
  Force_measured : Inport
  h_k : Inport  Port=2
  forget : Inport  Port=3
  Demux : Demux  Outputs=5
  MATLAB Function : MATLAB Function  TreatAsAtomicUnit=on
      settings: PermitHierarchicalResolution=ParametersOnly
  Memory1 : Memory
  Memory10 : Memory  X0=y_X
  Memory11 : Memory  X0=h_X_old
  Memory7 : Memory  X0=p_X
  Memory8 : Memory  X0=Pcov_X
  Memory9 : Memory  X0=y_X_est_old
  Selector : Selector  NumberOfDimensions=2  InputPortWidth=1  IndexOptions=Index vector (dialog),Index vector (dialog)  Indices=[1:5],1  OutputSizes=1,1
  Terminator : Terminator
  Time Scope : TimeScope  Commented=on  DefaultConfigurationName=spbscopes.TimeScopeBlockCfg  NumInputPorts=5
  force_est_latest : Outport
  force_est : Outport  Port=2
  force_measured : Outport  Port=3
  par_est : Outport  Port=4
  wires:
  Memory9/1 -> MATLAB Function/6("y_est_old ")
  MATLAB Function/1(P_cov) -> Memory8/1
  Memory10/1 -> MATLAB Function/5("y_old ")
  MATLAB Function/5(h_old) -> Memory11/1
  Memory11/1 -> MATLAB Function/7("h_old ")
  MATLAB Function/3(y_old) -> Memory10/1, force_measured/1
  Memory7/1 -> MATLAB Function/2("pk ")
  MATLAB Function/4(y_est_old) -> Memory9/1, force_est/1
  Memory8/1 -> MATLAB Function/1("P_cov ")
  MATLAB Function/2(pk) -> Selector/1, Memory7/1
  h_k/1 -> MATLAB Function/4(hk_new)
  Force_measured/1 -> MATLAB Function/3("y_new ")
  MATLAB Function/6(counter) -> Memory1/1
  Memory1/1 -> MATLAB Function/8("counter ")
  forget/1 -> MATLAB Function/9(forget)  "lambda"
  MATLAB Function/7(y_est) -> force_est_latest/1
  MATLAB Function/8(y_new) -> Terminator/1  "y_new putthrough"
  Selector/1 -> Demux/1, par_est/1
  Demux/2 -> Time Scope/2  "CXa"
  Demux/1 -> Time Scope/1  "CX0"
  Demux/3 -> Time Scope/3  "CXa2"
  Demux/5 -> Time Scope/5  "CXde"
  Demux/4 -> Time Scope/4  "CXq"

== system Citation_2015a/Aerodynamic Parameter Estimation/CY ==
  note: reset covariance matrix to initial condition one time. whenever a failure has been detected
  note: if lambda=1 => no forgetting
  note: counter is still obsolete
  Force_measured : Inport
  h_k : Inport  Port=2
  forget : Inport  Port=3
  fail : Inport  Port=4
  Constant : Constant  Value=Pcov_Y
  Demux : Demux  Outputs=6
  MATLAB Function : MATLAB Function  TreatAsAtomicUnit=on
      settings: PermitHierarchicalResolution=ParametersOnly
  Memory1 : Memory
  Memory10 : Memory  X0=y_Y
  Memory11 : Memory  X0=h_Y_old
  Memory7 : Memory  X0=p_Y
  Memory8 : Memory  X0=Pcov_Y
  Memory9 : Memory  X0=y_Y_est_old
  Selector : Selector  NumberOfDimensions=2  InputPortWidth=1  IndexOptions=Index vector (dialog),Index vector (dialog)  Indices=[1:6],1  OutputSizes=1,1
  Switch : Switch  Criteria=u2 > Threshold
  Terminator : Terminator
  Time Scope : TimeScope  Commented=on  DefaultConfigurationName=spbscopes.TimeScopeBlockCfg  NumInputPorts=6
  force_est_latest : Outport
  force_est : Outport  Port=2
  force_measured : Outport  Port=3
  par_est : Outport  Port=4
  wires:
  MATLAB Function/8(y_new) -> Terminator/1  "y_new putthrough"
  MATLAB Function/7(y_est) -> force_est_latest/1
  forget/1 -> MATLAB Function/9(forget)  "lambda"
  Memory1/1 -> MATLAB Function/8("counter ")
  MATLAB Function/6(counter) -> Memory1/1
  Force_measured/1 -> MATLAB Function/3("y_new ")
  h_k/1 -> MATLAB Function/4(hk_new)
  MATLAB Function/2(pk) -> Selector/1, Memory7/1
  Memory8/1 -> Switch/3
  MATLAB Function/4(y_est_old) -> force_est/1, Memory9/1
  Memory7/1 -> MATLAB Function/2("pk ")
  MATLAB Function/3(y_old) -> force_measured/1, Memory10/1
  Memory11/1 -> MATLAB Function/7("h_old ")
  MATLAB Function/5(h_old) -> Memory11/1
  Memory10/1 -> MATLAB Function/5("y_old ")
  MATLAB Function/1(P_cov) -> Memory8/1
  Memory9/1 -> MATLAB Function/6("y_est_old ")
  fail/1 -> Switch/2
  Constant/1 -> Switch/1
  Switch/1 -> MATLAB Function/1("P_cov ")
  Selector/1 -> Demux/1, par_est/1
  Demux/2 -> Time Scope/2  "CYB"
  Demux/1 -> Time Scope/1  "CY0"
  Demux/3 -> Time Scope/3  "CYp"
  Demux/4 -> Time Scope/4  "CYr"
  Demux/5 -> Time Scope/5  "CYda"
  Demux/6 -> Time Scope/6  "CYdr"

== system Citation_2015a/Aerodynamic Parameter Estimation/CZ ==
  note: counter is still obsolete
  note: if lambda=1 => no forgetting
  Force_measured : Inport
  h_k : Inport  Port=2
  forget : Inport  Port=3
  Demux : Demux
  MATLAB Function : MATLAB Function  TreatAsAtomicUnit=on
      settings: PermitHierarchicalResolution=ParametersOnly
  Memory1 : Memory
  Memory10 : Memory  X0=y_Z
  Memory11 : Memory  X0=h_Z_old
  Memory7 : Memory  X0=p_Z
  Memory8 : Memory  X0=Pcov_Z
  Memory9 : Memory  X0=y_Z_est_old
  Selector : Selector  NumberOfDimensions=2  InputPortWidth=1  IndexOptions=Index vector (dialog),Index vector (dialog)  Indices=[1:4],1  OutputSizes=1,1
  Terminator : Terminator
  Time Scope : TimeScope  Commented=on  DefaultConfigurationName=spbscopes.TimeScopeBlockCfg  NumInputPorts=4
  force_est_latest : Outport
  force_est : Outport  Port=2
  force_measured : Outport  Port=3
  par_est : Outport  Port=4
  wires:
  Memory9/1 -> MATLAB Function/6("y_est_old ")
  MATLAB Function/1(P_cov) -> Memory8/1
  Memory10/1 -> MATLAB Function/5("y_old ")
  MATLAB Function/5(h_old) -> Memory11/1
  Memory11/1 -> MATLAB Function/7("h_old ")
  MATLAB Function/3(y_old) -> Memory10/1, force_measured/1
  Memory7/1 -> MATLAB Function/2("pk ")
  MATLAB Function/4(y_est_old) -> Memory9/1, force_est/1
  Memory8/1 -> MATLAB Function/1("P_cov ")
  MATLAB Function/2(pk) -> Memory7/1, Selector/1
  h_k/1 -> MATLAB Function/4(hk_new)
  Force_measured/1 -> MATLAB Function/3("y_new ")
  MATLAB Function/6(counter) -> Memory1/1
  Memory1/1 -> MATLAB Function/8("counter ")
  forget/1 -> MATLAB Function/9(forget)  "lambda"
  MATLAB Function/7(y_est) -> force_est_latest/1
  MATLAB Function/8(y_new) -> Terminator/1  "y_new putthrough"
  Selector/1 -> Demux/1, par_est/1
  Demux/1 -> Time Scope/1  "CZ0"
  Demux/2 -> Time Scope/2  "CZa"
  Demux/3 -> Time Scope/3  "CZq"
  Demux/4 -> Time Scope/4  "CZde"

== system Citation_2015a/Aerodynamic Parameter Estimation/Cl ==
  note: if lambda=1 => no forgetting
  Force_measured : Inport
  h_k : Inport  Port=2
  forget : Inport  Port=3
  "fail " : Inport  Port=4
  Constant : Constant  Value=Pcov_l
  MATLAB Function : MATLAB Function  TreatAsAtomicUnit=on
      settings: PermitHierarchicalResolution=ParametersOnly
  Memory10 : Memory  X0=y_l
  Memory11 : Memory  X0=h_l_old
  Memory7 : Memory  X0=p_l
  Memory8 : Memory  X0=Pcov_l
  Memory9 : Memory  X0=y_l_est_old
  Selector : Selector  NumberOfDimensions=2  InputPortWidth=1  IndexOptions=Index vector (dialog),Index vector (dialog)  Indices=[1:6],1  OutputSizes=1,1
  Switch : Switch  Criteria=u2 > Threshold
  force_est_latest : Outport
  force_est : Outport  Port=2
  force_measured : Outport  Port=3
  par_est_latest : Outport  Port=4
  par_est : Outport  Port=5
  wires:
  MATLAB Function/6(y_est) -> force_est_latest/1
  forget/1 -> MATLAB Function/8(forget)  "lambda"
  Force_measured/1 -> MATLAB Function/3(y_new)
  h_k/1 -> MATLAB Function/4(hk_new)
  MATLAB Function/2(pk) -> par_est/1, Selector/1, Memory7/1
  MATLAB Function/4(y_est_old) -> Memory9/1, force_est/1
  Memory7/1 -> MATLAB Function/2("pk ")
  MATLAB Function/3(y_old) -> Memory10/1, force_measured/1
  Memory11/1 -> MATLAB Function/7("h_old ")
  MATLAB Function/5(h_old) -> Memory11/1
  Memory10/1 -> MATLAB Function/5("y_old ")
  MATLAB Function/1(P_cov) -> Memory8/1
  Memory9/1 -> MATLAB Function/6("y_est_old ")
  "fail "/1 -> Switch/2
  Constant/1 -> Switch/1
  Memory8/1 -> Switch/3
  Switch/1 -> MATLAB Function/1("P_cov ")
  Selector/1 -> par_est_latest/1

== system Citation_2015a/Aerodynamic Parameter Estimation/Cm ==
  note: counter is still obsolete
  note: if lambda=1 => no forgetting
  Force_measured : Inport
  h_k : Inport  Port=2
  forget : Inport  Port=3
  Demux : Demux
  MATLAB Function : MATLAB Function  TreatAsAtomicUnit=on
      settings: PermitHierarchicalResolution=ParametersOnly
  Memory1 : Memory
  Memory10 : Memory  X0=y_m
  Memory11 : Memory  X0=h_m_old
  Memory7 : Memory  X0=p_m
  Memory8 : Memory  X0=Pcov_m
  Memory9 : Memory  X0=y_m_est_old
  Selector : Selector  NumberOfDimensions=2  InputPortWidth=1  IndexOptions=Index vector (dialog),Index vector (dialog)  Indices=[1:4],1  OutputSizes=1,1
  Terminator : Terminator
  Time Scope : TimeScope  Commented=on  DefaultConfigurationName=spbscopes.TimeScopeBlockCfg  NumInputPorts=4
  force_est_latest : Outport
  force_est : Outport  Port=2
  force_measured : Outport  Port=3
  par_est : Outport  Port=4
  wires:
  Memory9/1 -> MATLAB Function/6("y_est_old ")
  MATLAB Function/1(P_cov) -> Memory8/1
  Memory10/1 -> MATLAB Function/5("y_old ")
  MATLAB Function/5(h_old) -> Memory11/1
  Memory11/1 -> MATLAB Function/7("h_old ")
  MATLAB Function/3(y_old) -> Memory10/1, force_measured/1
  Memory7/1 -> MATLAB Function/2("pk ")
  MATLAB Function/4(y_est_old) -> Memory9/1, force_est/1
  Memory8/1 -> MATLAB Function/1("P_cov ")
  MATLAB Function/2(pk) -> Selector/1, Memory7/1
  h_k/1 -> MATLAB Function/4(hk_new)
  Force_measured/1 -> MATLAB Function/3("y_new ")
  MATLAB Function/6(counter) -> Memory1/1
  Memory1/1 -> MATLAB Function/8("counter ")
  forget/1 -> MATLAB Function/9(forget)  "lambda"
  MATLAB Function/7(y_est) -> force_est_latest/1
  MATLAB Function/8(y_new) -> Terminator/1  "y_new putthrough"
  Selector/1 -> Demux/1, par_est/1
  Demux/4 -> Time Scope/4  "Cmde"
  Demux/3 -> Time Scope/3  "Cmq"
  Demux/2 -> Time Scope/2  "Cma"
  Demux/1 -> Time Scope/1  "Cm0"

== system Citation_2015a/Aerodynamic Parameter Estimation/Cn ==
  note: if lambda=1 => no forgetting
  note: counter is still obsolete
  Force_measured : Inport
  h_k : Inport  Port=2
  forget : Inport  Port=3
  "fail " : Inport  Port=4
  Constant : Constant  Value=Pcov_n
  Demux : Demux  Outputs=6
  MATLAB Function : MATLAB Function  TreatAsAtomicUnit=on
      settings: PermitHierarchicalResolution=ParametersOnly
  Memory1 : Memory
  Memory10 : Memory  X0=y_n
  Memory11 : Memory  X0=h_n_old
  Memory7 : Memory  X0=p_n
  Memory8 : Memory  X0=Pcov_n
  Memory9 : Memory  X0=y_n_est_old
  Selector : Selector  NumberOfDimensions=2  InputPortWidth=1  IndexOptions=Index vector (dialog),Index vector (dialog)  Indices=[1:6],1  OutputSizes=1,1
  Switch : Switch  Criteria=u2 > Threshold
  Terminator : Terminator
  Time Scope : TimeScope  Commented=on  DefaultConfigurationName=spbscopes.TimeScopeBlockCfg  NumInputPorts=6
  force_est_latest : Outport
  force_est : Outport  Port=2
  force_measured : Outport  Port=3
  par_est : Outport  Port=4
  wires:
  MATLAB Function/8(y_new) -> Terminator/1  "y_new putthrough"
  MATLAB Function/7(y_est) -> force_est_latest/1
  forget/1 -> MATLAB Function/9(forget)  "lambda"
  Memory1/1 -> MATLAB Function/8("counter ")
  MATLAB Function/6(counter) -> Memory1/1
  Force_measured/1 -> MATLAB Function/3("y_new ")
  h_k/1 -> MATLAB Function/4(hk_new)
  MATLAB Function/2(pk) -> Selector/1, Memory7/1
  MATLAB Function/4(y_est_old) -> force_est/1, Memory9/1
  Memory7/1 -> MATLAB Function/2("pk ")
  MATLAB Function/3(y_old) -> force_measured/1, Memory10/1
  Memory11/1 -> MATLAB Function/7("h_old ")
  MATLAB Function/5(h_old) -> Memory11/1
  Memory10/1 -> MATLAB Function/5("y_old ")
  MATLAB Function/1(P_cov) -> Memory8/1
  Memory9/1 -> MATLAB Function/6("y_est_old ")
  "fail "/1 -> Switch/2
  Constant/1 -> Switch/1
  Memory8/1 -> Switch/3
  Switch/1 -> MATLAB Function/1("P_cov ")
  Selector/1 -> par_est/1, Demux/1
  Demux/1 -> Time Scope/1  "Cn0"
  Demux/2 -> Time Scope/2  "CnB"
  Demux/3 -> Time Scope/3  "Cnp"
  Demux/4 -> Time Scope/4  "Cnr"
  Demux/5 -> Time Scope/5  "Cnda"
  Demux/6 -> Time Scope/6  "Cndr"

== system Citation_2015a/Aerodynamic Parameter Estimation/Failure monitor system  ==
  note: variance
      | sigma_avg
      | sigma_avg
      | moving average
      | AutoCorr
      | AutoCorr_avg
  Stat_Y : Inport
  Stat_l : Inport  Port=2
  Stat_n : Inport  Port=3
  Demux1 : Demux  Commented=on  Outputs=6
  Demux2 : Demux  Outputs=[3 1 2]
  Demux3 : Demux  Commented=on  Outputs=6
  Fcn : Fcn  Expr=u>movavg_thresh
  MATLAB Function : MATLAB Function  TreatAsAtomicUnit=on
      settings: PermitHierarchicalResolution=ParametersOnly
  Memory : Memory
  Send message : Subsystem  TreatAsAtomicUnit=on
  Terminator : Terminator
  Terminator1 : Terminator
  Time Scope3 : TimeScope  Commented=on  DefaultConfigurationName=spbscopes.TimeScopeBlockCfg  NumInputPorts=2
  Y : TimeScope  Commented=on  DefaultConfigurationName=spbscopes.TimeScopeBlockCfg  NumInputPorts=3
  Yn : TimeScope  Commented=on  DefaultConfigurationName=spbscopes.TimeScopeBlockCfg  NumInputPorts=3
  fail_detect : Outport
  wires:
  Demux1/4 -> Y/2  "moving avg Y"
  Stat_Y/1 -> Demux1/1
  Demux1/1 -> Y/1  "variance Y"
  Demux1/5 -> Y/3  "Autocorr Y"
  Stat_l/1 -> Demux2/1
  Demux2/2 -> Time Scope3/2, Fcn/1  "moving avg l"
  Demux3/4 -> Yn/2  "moving avg n"
  Stat_n/1 -> Demux3/1
  Demux3/1 -> Yn/1  "variance n"
  Demux3/5 -> Yn/3  "Autocorr n"
  Fcn/1 -> MATLAB Function/1(u)
  MATLAB Function/1(y) -> fail_detect/1, Time Scope3/1, Send message/Trigger  "fail detect pulse"
  MATLAB Function/2(counter) -> Memory/1
  Memory/1 -> MATLAB Function/2("counter ")
  Demux2/1 -> Terminator/1  "variance l"
  Demux2/3 -> Terminator1/1

== system Citation_2015a/Aerodynamic Parameter Estimation/Statistics 2 ==
  note: variance
      | sigma_avg
      | sigma_avg
      | moving average
      | AutoCorr
      | AutoCorr_avg
  Force : Inport
  ForceEstLatest : Inport  Port=2
  ForceEstWindow : Inport  Port=3
  ForceWindow : Inport  Port=4
  "kgap " : Inport  Port=5
  Auto_correlation : Subsystem
  Floor : Rounding
  Mux : Mux  Inputs=5
  Sum : Sum  Inputs=|-+
  Sum1 : Sum  Inputs=|+-
  moving average square : MATLAB Function  TreatAsAtomicUnit=on
      settings: PermitHierarchicalResolution=ParametersOnly
  variance : Subsystem
  statistics : Outport
  wires:
  Sum/1 -> Auto_correlation/1(delta_window), moving average square/1(delta)
  Sum1/1 -> variance/1(delta)  "delta"
  "kgap "/1 -> Floor/1
  Floor/1 -> Auto_correlation/2(kgap)
  ForceWindow/1 -> Sum/2
  ForceEstWindow/1 -> Sum/1
  ForceEstLatest/1 -> Sum1/2
  Force/1 -> Sum1/1
  variance/1(variance) -> Mux/1
  variance/2(sigma_avg) -> Mux/2
  moving average square/1(av) -> Mux/3
  Auto_correlation/1(PI_kgap) -> Mux/4
  Auto_correlation/2(PI_kgap_avg) -> Mux/5
  Mux/1 -> statistics/1

== system Citation_2015a/Aerodynamic Parameter Estimation/Statistics 3 ==
  note: variance
      | sigma_avg
      | sigma_avg
      | moving average
      | AutoCorr
      | AutoCorr_avg
  Force : Inport
  ForceEstLatest : Inport  Port=2
  ForceEstWindow : Inport  Port=3
  ForceWindow : Inport  Port=4
  "kgap " : Inport  Port=5
  Auto_correlation : Subsystem
  Floor : Rounding
  Mux : Mux  Inputs=5
  Sum : Sum  Inputs=|-+
  Sum1 : Sum  Inputs=|+-
  Time Scope : TimeScope  Commented=on  DefaultConfigurationName=spbscopes.TimeScopeBlockCfg  NumInputPorts=3
  Time Scope1 : TimeScope  Commented=on  DefaultConfigurationName=spbscopes.TimeScopeBlockCfg
  moving average square : MATLAB Function  TreatAsAtomicUnit=on
      settings: PermitHierarchicalResolution=ParametersOnly
  variance : Subsystem
  statistics : Outport
  wires:
  Mux/1 -> statistics/1
  Auto_correlation/2(PI_kgap_avg) -> Mux/5
  Auto_correlation/1(PI_kgap) -> Time Scope/3, Mux/4  "auto correlation"
  moving average square/1(av) -> Time Scope1/1, Time Scope/2, Mux/3  "moving square average"
  variance/2(sigma_avg) -> Mux/2
  variance/1(variance) -> Time Scope/1, Mux/1  "variance"
  Force/1 -> Sum1/1
  ForceEstLatest/1 -> Sum1/2
  ForceEstWindow/1 -> Sum/1
  ForceWindow/1 -> Sum/2
  Floor/1 -> Auto_correlation/2(kgap)
  "kgap "/1 -> Floor/1
  Sum1/1 -> variance/1(delta)  "delta"
  Sum/1 -> moving average square/1(delta), Auto_correlation/1(delta_window)

== system Citation_2015a/Aerodynamic Parameter Estimation/Statistics 4 ==
  note: variance
      | sigma_avg
      | sigma_avg
      | moving average
      | AutoCorr
      | AutoCorr_avg
  Force : Inport
  ForceEstLatest : Inport  Port=2
  ForceEstWindow : Inport  Port=3
  ForceWindow : Inport  Port=4
  "kgap " : Inport  Port=5
  Auto_correlation : Subsystem
  Floor : Rounding
  Mux : Mux  Inputs=5
  Sum : Sum  Inputs=|-+
  Sum1 : Sum  Inputs=|+-
  moving average square : MATLAB Function  TreatAsAtomicUnit=on
      settings: PermitHierarchicalResolution=ParametersOnly
  variance : Subsystem
  statistics : Outport
  wires:
  Sum/1 -> Auto_correlation/1(delta_window), moving average square/1(delta)
  Sum1/1 -> variance/1(delta)  "delta"
  "kgap "/1 -> Floor/1
  Floor/1 -> Auto_correlation/2(kgap)
  ForceWindow/1 -> Sum/2
  ForceEstWindow/1 -> Sum/1
  ForceEstLatest/1 -> Sum1/2
  Force/1 -> Sum1/1
  variance/1(variance) -> Mux/1
  variance/2(sigma_avg) -> Mux/2
  moving average square/1(av) -> Mux/3
  Auto_correlation/1(PI_kgap) -> Mux/4
  Auto_correlation/2(PI_kgap_avg) -> Mux/5
  Mux/1 -> statistics/1
